simulink model "Quadrotor"  (R2022b)
settings: Solver=FixedStepAuto  StartTime=0.0  StopTime=1000  FixedStep=0.0005  RelTol=1e-3
model workspace (MAT data in the model file):
  b = 0.000142
  g = 9.8
  m = 1
undefined symbols (not defined in the file): Pitch, Roll, X, Y, Yaw, Z
libraries: simulink x12, slpidlib x9, sharedtransform x1, uavutilslib x1, aerolibanim x1
(part 2 of 3)

== system Quadrotor/Attitude Loop(PD)/P&R ==
  Pitch_d : Inport
  Roll_d : Inport  Port=2
  Pitch : Inport  Port=3
  Roll : Inport  Port=4
  PID Controller P : slpidlib/PID Controller  Controller=PD  Form=Parallel  TimeDomain=Continuous-time  UseExternalTs=off  SampleTime=-1  IntegratorMethod=Forward Euler  FilterMethod=Forward Euler  ControllerParametersSource=internal  P=0.002  I=1.51679966097293e-05  UseKiTs=off  D=0.004  N=3.58143563707461  UseFilter=on  TunerSelectOption=Transfer Function Based (PID Tuner App)  InitialConditionSource=internal  InitialConditionForIntegrator=0  InitialConditionForFilter=0  DifferentiatorICPrevScaledInput=0  ExternalReset=none  TrackingMode=off  Kt=1  LimitOutput=off  SatLimitsSource=internal  UpperSaturationLimit=inf  LowerSaturationLimit=-inf  LinearizeAsGain=on  AntiWindupMode=none  Kb=1  LimitIntegrator=off  UpperIntegratorSaturationLimit=inf  LowerIntegratorSaturationLimit=-inf  POutMin=[]  POutMax=[]  IOutMin=[]  IOutMax=[]  DOutMin=[]  DOutMax=[]  NOutMin=[]  NOutMax=[]  SumOutMin=[]  SumOutMax=[]  SaturationOutMin=[]  SaturationOutMax=[]  PParamMin=[]  PParamMax=[]  IParamMin=[]  IParamMax=[]  DParamMin=[]  DParamMax=[]  NParamMin=[]  NParamMax=[]  KbParamMin=[]  KbParamMax=[]  KtParamMin=[]  KtParamMax=[]  KbOutMin=[]  KbOutMax=[]  KtOutMin=[]  KtOutMax=[]  IntegratorOutMin=[]  IntegratorOutMax=[]  FilterOutMin=[]  FilterOutMax=[]  SumI1OutMin=[]  SumI1OutMax=[]  SumI2OutMin=[]  SumI2OutMax=[]  SumI3OutMin=[]  SumI3OutMax=[]  SumI4OutMin=[]  SumI4OutMax=[]  SumDOutMin=[]  SumDOutMax=[]  DifferentiatorOutMin=[]  DifferentiatorOutMax=[]  FilterDiffOutCoefMin=[]  FilterDiffOutCoefMax=[]  ReciprocalOutMin=[]  ReciprocalOutMax=[]  SumDenOutMin=[]  SumDenOutMax=[]  SumNumOutMin=[]  SumNumOutMax=[]  DivideOutMin=[]  DivideOutMax=[]  UdiffTsProdOutMin=[]  UdiffTsProdOutMax=[]  NTsProdOutMin=[]  NTsProdOutMax=[]  UintegralTsProdOutMin=[]  UintegralTsProdOutMax=[]  UngainTsProdOutMin=[]  UngainTsProdOutMax=[]  ClampingZeroOutDataTypeStr=Inherit: Inherit via back propagation  ClampingZeroOutMin=[]  ClampingZeroOutMax=[]  FilterDenConstantOutDataTypeStr=Inherit: Inherit via back propagation  FilterDenConstantOutMin=[]  FilterDenConstantOutMax=[]  PCopyOutDataTypeStr=Inherit: Inherit via back propagation  PCopyOutMin=[]  PCopyOutMax=[]  NCopyOutDataTypeStr=Inherit: Inherit via back propagation  NCopyOutMin=[]  NCopyOutMax=[]  IntegratorContinuousStateAttributes=''  IntegratorStateMustResolveToSignalObject=off  IntegratorRTWStateStorageClass=Auto  FilterContinuousStateAttributes=''  FilterStateMustResolveToSignalObject=off  FilterRTWStateStorageClass=Auto  ParallelPVariant=InternalParameters  IdealPVariant=Disabled  IVariant=Disabled  DVariant=InternalParameters  IntegratorVariant=Disabled  SatVariant=Disabled  AWVariant=Disabled  PCopyVariant=Disabled  TRVariant=Disabled  FdbkBlocksVariant=Forward  IdealPFdbkVariant=Disabled  SatFdbkVariant=Disabled  DerivativeFilterVariant=ContFilter  NVariant=InternalParameters  NCopyVariant=Disabled  FilterICVariant=InternalICsFilter  IntegratorICVariant=Disabled  ExternalResetVariant=Disabled  TRSumVariant=Passthrough  SumFdbkVariant=Disabled  SumVariant=Sum_PD  TsampFilterVariant=InternalTs  TsampNgainVariant=Passthrough  TsampIntegralVariant=Disabled_SignalSpec  ExternalSaturationOutDataTypeStr=Inherit: Same as second input
  PID Controller R : slpidlib/PID Controller  Controller=PD  Form=Parallel  TimeDomain=Continuous-time  UseExternalTs=off  SampleTime=-1  IntegratorMethod=Forward Euler  FilterMethod=Forward Euler  ControllerParametersSource=internal  P=0.000517944009365722  I=2.09015293720685e-05  UseKiTs=off  D=0.0031516571893313  N=4.69883432592557  UseFilter=on  TunerSelectOption=Transfer Function Based (PID Tuner App)  InitialConditionSource=internal  InitialConditionForIntegrator=0  InitialConditionForFilter=0  DifferentiatorICPrevScaledInput=0  ExternalReset=none  TrackingMode=off  Kt=1  LimitOutput=off  SatLimitsSource=internal  UpperSaturationLimit=inf  LowerSaturationLimit=-inf  LinearizeAsGain=on  AntiWindupMode=none  Kb=1  LimitIntegrator=off  UpperIntegratorSaturationLimit=inf  LowerIntegratorSaturationLimit=-inf  POutMin=[]  POutMax=[]  IOutMin=[]  IOutMax=[]  DOutMin=[]  DOutMax=[]  NOutMin=[]  NOutMax=[]  SumOutMin=[]  SumOutMax=[]  SaturationOutMin=[]  SaturationOutMax=[]  PParamMin=[]  PParamMax=[]  IParamMin=[]  IParamMax=[]  DParamMin=[]  DParamMax=[]  NParamMin=[]  NParamMax=[]  KbParamMin=[]  KbParamMax=[]  KtParamMin=[]  KtParamMax=[]  KbOutMin=[]  KbOutMax=[]  KtOutMin=[]  KtOutMax=[]  IntegratorOutMin=[]  IntegratorOutMax=[]  FilterOutMin=[]  FilterOutMax=[]  SumI1OutMin=[]  SumI1OutMax=[]  SumI2OutMin=[]  SumI2OutMax=[]  SumI3OutMin=[]  SumI3OutMax=[]  SumI4OutMin=[]  SumI4OutMax=[]  SumDOutMin=[]  SumDOutMax=[]  DifferentiatorOutMin=[]  DifferentiatorOutMax=[]  FilterDiffOutCoefMin=[]  FilterDiffOutCoefMax=[]  ReciprocalOutMin=[]  ReciprocalOutMax=[]  SumDenOutMin=[]  SumDenOutMax=[]  SumNumOutMin=[]  SumNumOutMax=[]  DivideOutMin=[]  DivideOutMax=[]  UdiffTsProdOutMin=[]  UdiffTsProdOutMax=[]  NTsProdOutMin=[]  NTsProdOutMax=[]  UintegralTsProdOutMin=[]  UintegralTsProdOutMax=[]  UngainTsProdOutMin=[]  UngainTsProdOutMax=[]  ClampingZeroOutDataTypeStr=Inherit: Inherit via back propagation  ClampingZeroOutMin=[]  ClampingZeroOutMax=[]  FilterDenConstantOutDataTypeStr=Inherit: Inherit via back propagation  FilterDenConstantOutMin=[]  FilterDenConstantOutMax=[]  PCopyOutDataTypeStr=Inherit: Inherit via back propagation  PCopyOutMin=[]  PCopyOutMax=[]  NCopyOutDataTypeStr=Inherit: Inherit via back propagation  NCopyOutMin=[]  NCopyOutMax=[]  IntegratorContinuousStateAttributes=''  IntegratorStateMustResolveToSignalObject=off  IntegratorRTWStateStorageClass=Auto  FilterContinuousStateAttributes=''  FilterStateMustResolveToSignalObject=off  FilterRTWStateStorageClass=Auto  ParallelPVariant=InternalParameters  IdealPVariant=Disabled  IVariant=Disabled  DVariant=InternalParameters  IntegratorVariant=Disabled  SatVariant=Disabled  AWVariant=Disabled  PCopyVariant=Disabled  TRVariant=Disabled  FdbkBlocksVariant=Forward  IdealPFdbkVariant=Disabled  SatFdbkVariant=Disabled  DerivativeFilterVariant=ContFilter  NVariant=InternalParameters  NCopyVariant=Disabled  FilterICVariant=InternalICsFilter  IntegratorICVariant=Disabled  ExternalResetVariant=Disabled  TRSumVariant=Passthrough  SumFdbkVariant=Disabled  SumVariant=Sum_PD  TsampFilterVariant=InternalTs  TsampNgainVariant=Passthrough  TsampIntegralVariant=Disabled_SignalSpec  ExternalSaturationOutDataTypeStr=Inherit: Same as second input
  Sum5 : Sum  Inputs=|+-
  Sum6 : Sum  Inputs=|+-
  U3 : Outport
  U2 : Outport  Port=2
  wires:
  PID Controller P/1 -> U3/1
  Pitch/1 -> Sum5/2
  Sum6/1 -> PID Controller R/1
  Sum5/1 -> PID Controller P/1
  Roll/1 -> Sum6/2
  PID Controller R/1 -> U2/1
  Pitch_d/1 -> Sum5/1
  Roll_d/1 -> Sum6/1

== system Quadrotor/Attitude Loop(PD)/yaw ==
  Yaw_d : Inport
  Yaw : Inport  Port=2
  PID Controller Y : slpidlib/PID Controller  Controller=PD  Form=Parallel  TimeDomain=Continuous-time  UseExternalTs=off  SampleTime=-1  IntegratorMethod=Forward Euler  FilterMethod=Forward Euler  ControllerParametersSource=internal  P=0.00070917828540938  I=0  UseKiTs=off  D=0.00337767414842328  N=2.26407668868773  UseFilter=on  TunerSelectOption=Transfer Function Based (PID Tuner App)  InitialConditionSource=internal  InitialConditionForIntegrator=0  InitialConditionForFilter=0  DifferentiatorICPrevScaledInput=0  ExternalReset=none  TrackingMode=off  Kt=1  LimitOutput=off  SatLimitsSource=internal  UpperSaturationLimit=inf  LowerSaturationLimit=-inf  LinearizeAsGain=on  AntiWindupMode=none  Kb=1  LimitIntegrator=off  UpperIntegratorSaturationLimit=inf  LowerIntegratorSaturationLimit=-inf  POutMin=[]  POutMax=[]  IOutMin=[]  IOutMax=[]  DOutMin=[]  DOutMax=[]  NOutMin=[]  NOutMax=[]  SumOutMin=[]  SumOutMax=[]  SaturationOutMin=[]  SaturationOutMax=[]  PParamMin=[]  PParamMax=[]  IParamMin=[]  IParamMax=[]  DParamMin=[]  DParamMax=[]  NParamMin=[]  NParamMax=[]  KbParamMin=[]  KbParamMax=[]  KtParamMin=[]  KtParamMax=[]  KbOutMin=[]  KbOutMax=[]  KtOutMin=[]  KtOutMax=[]  IntegratorOutMin=[]  IntegratorOutMax=[]  FilterOutMin=[]  FilterOutMax=[]  SumI1OutMin=[]  SumI1OutMax=[]  SumI2OutMin=[]  SumI2OutMax=[]  SumI3OutMin=[]  SumI3OutMax=[]  SumI4OutMin=[]  SumI4OutMax=[]  SumDOutMin=[]  SumDOutMax=[]  DifferentiatorOutMin=[]  DifferentiatorOutMax=[]  FilterDiffOutCoefMin=[]  FilterDiffOutCoefMax=[]  ReciprocalOutMin=[]  ReciprocalOutMax=[]  SumDenOutMin=[]  SumDenOutMax=[]  SumNumOutMin=[]  SumNumOutMax=[]  DivideOutMin=[]  DivideOutMax=[]  UdiffTsProdOutMin=[]  UdiffTsProdOutMax=[]  NTsProdOutMin=[]  NTsProdOutMax=[]  UintegralTsProdOutMin=[]  UintegralTsProdOutMax=[]  UngainTsProdOutMin=[]  UngainTsProdOutMax=[]  ClampingZeroOutDataTypeStr=Inherit: Inherit via back propagation  ClampingZeroOutMin=[]  ClampingZeroOutMax=[]  FilterDenConstantOutDataTypeStr=Inherit: Inherit via back propagation  FilterDenConstantOutMin=[]  FilterDenConstantOutMax=[]  PCopyOutDataTypeStr=Inherit: Inherit via back propagation  PCopyOutMin=[]  PCopyOutMax=[]  NCopyOutDataTypeStr=Inherit: Inherit via back propagation  NCopyOutMin=[]  NCopyOutMax=[]  IntegratorContinuousStateAttributes=''  IntegratorStateMustResolveToSignalObject=off  IntegratorRTWStateStorageClass=Auto  FilterContinuousStateAttributes=''  FilterStateMustResolveToSignalObject=off  FilterRTWStateStorageClass=Auto  ParallelPVariant=InternalParameters  IdealPVariant=Disabled  IVariant=Disabled  DVariant=InternalParameters  IntegratorVariant=Disabled  SatVariant=Disabled  AWVariant=Disabled  PCopyVariant=Disabled  TRVariant=Disabled  FdbkBlocksVariant=Forward  IdealPFdbkVariant=Disabled  SatFdbkVariant=Disabled  DerivativeFilterVariant=ContFilter  NVariant=InternalParameters  NCopyVariant=Disabled  FilterICVariant=InternalICsFilter  IntegratorICVariant=Disabled  ExternalResetVariant=Disabled  TRSumVariant=Passthrough  SumFdbkVariant=Disabled  SumVariant=Sum_PD  TsampFilterVariant=InternalTs  TsampNgainVariant=Passthrough  TsampIntegralVariant=Disabled_SignalSpec  ExternalSaturationOutDataTypeStr=Inherit: Same as second input
  Sum2 : Sum  Inputs=|+-
  U4 : Outport
  wires:
  Yaw/1 -> Sum2/2
  Sum2/1 -> PID Controller Y/1
  Yaw_d/1 -> Sum2/1
  PID Controller Y/1 -> U4/1

== system Quadrotor/Demand_LADRC/generate ==
  butterfly : Subsystem
  circle 500 : Subsystem
  ramp 30 : Subsystem
  screw 600 : Subsystem
  steady1 : Subsystem
  up 30 : Subsystem
  up : Outport
  ramp : Outport  Port=2
  circle : Outport  Port=3
  screw : Outport  Port=4
  butterfiy : Outport  Port=5
  steady : Outport  Port=6
  wires:
  screw 600/1(Out1) -> screw/1
  butterfly/1(Out1) -> butterfiy/1
  circle 500/1(Out1) -> circle/1
  ramp 30/1(Out1) -> ramp/1
  up 30/1(Out1) -> up/1
  steady1/1(Out1) -> steady/1

== system Quadrotor/Demand_LADRC/out ==
  In1 : Inport
  Bus Selector : BusSelector  OutputSignals=signal1,signal2,signal3,signal4
  To Workspace : ToWorkspace  VariableName=demand1  SampleTime=-1
  X_d : Outport
  Y_d : Outport  Port=2
  Z_d : Outport  Port=3
  Yaw_d : Outport  Port=4
  wires:
  Bus Selector/3 -> Z_d/1  "<signal3>"
  Bus Selector/2 -> Y_d/1  "<signal2>"
  Bus Selector/1 -> X_d/1  "<signal1>"
  Bus Selector/4 -> Yaw_d/1  "<signal4>"
  In1/1 -> To Workspace/1, Bus Selector/1

== system Quadrotor/Demand_PID/generate ==
  butterfly : Subsystem
  circle 500 : Subsystem
  ramp 30 : Subsystem
  screw 600 : Subsystem
  steady1 : Subsystem
  up 30 : Subsystem
  up : Outport
  ramp : Outport  Port=2
  circle : Outport  Port=3
  screw : Outport  Port=4
  butterfiy : Outport  Port=5
  steady : Outport  Port=6
  wires:
  screw 600/1(Out1) -> screw/1
  butterfly/1(Out1) -> butterfiy/1
  circle 500/1(Out1) -> circle/1
  ramp 30/1(Out1) -> ramp/1
  up 30/1(Out1) -> up/1
  steady1/1(Out1) -> steady/1

== system Quadrotor/Demand_PID/out ==
  In1 : Inport
  Bus Selector : BusSelector  OutputSignals=signal1,signal2,signal3,signal4
  To Workspace : ToWorkspace  VariableName=demand  SampleTime=-1
  X_d : Outport
  Y_d : Outport  Port=2
  Z_d : Outport  Port=3
  Yaw_d : Outport  Port=4
  wires:
  Bus Selector/3 -> Z_d/1  "<signal3>"
  Bus Selector/2 -> Y_d/1  "<signal2>"
  Bus Selector/1 -> X_d/1  "<signal1>"
  Bus Selector/4 -> Yaw_d/1  "<signal4>"
  In1/1 -> To Workspace/1, Bus Selector/1

== system Quadrotor/Formation Control/height ==
  Z_d : Inport
  Z : Inport  Port=2
  Constant : Constant  Value=g
  PID Controller Z : slpidlib/PID Controller  Controller=PID  Form=Parallel  TimeDomain=Discrete-time  UseExternalTs=off  SampleTime=-1  IntegratorMethod=Forward Euler  FilterMethod=Forward Euler  ControllerParametersSource=internal  P=3.53804542303513  I=0.723013447865675  UseKiTs=off  D=4.25131927818495  N=23.8074436453229  UseFilter=on  TunerSelectOption=Transfer Function Based (PID Tuner App)  InitialConditionSource=internal  InitialConditionForIntegrator=0  InitialConditionForFilter=0  DifferentiatorICPrevScaledInput=0  ExternalReset=none  TrackingMode=off  Kt=1  LimitOutput=off  SatLimitsSource=internal  UpperSaturationLimit=inf  LowerSaturationLimit=-inf  LinearizeAsGain=on  AntiWindupMode=none  Kb=1  LimitIntegrator=off  UpperIntegratorSaturationLimit=inf  LowerIntegratorSaturationLimit=-inf  POutMin=[]  POutMax=[]  IOutMin=[]  IOutMax=[]  DOutMin=[]  DOutMax=[]  NOutMin=[]  NOutMax=[]  SumOutMin=[]  SumOutMax=[]  SaturationOutMin=[]  SaturationOutMax=[]  PParamMin=[]  PParamMax=[]  IParamMin=[]  IParamMax=[]  DParamMin=[]  DParamMax=[]  NParamMin=[]  NParamMax=[]  KbParamMin=[]  KbParamMax=[]  KtParamMin=[]  KtParamMax=[]  KbOutMin=[]  KbOutMax=[]  KtOutMin=[]  KtOutMax=[]  IntegratorOutMin=[]  IntegratorOutMax=[]  FilterOutMin=[]  FilterOutMax=[]  SumI1OutMin=[]  SumI1OutMax=[]  SumI2OutMin=[]  SumI2OutMax=[]  SumI3OutMin=[]  SumI3OutMax=[]  SumI4OutMin=[]  SumI4OutMax=[]  SumDOutMin=[]  SumDOutMax=[]  DifferentiatorOutMin=[]  DifferentiatorOutMax=[]  FilterDiffOutCoefMin=[]  FilterDiffOutCoefMax=[]  ReciprocalOutMin=[]  ReciprocalOutMax=[]  SumDenOutMin=[]  SumDenOutMax=[]  SumNumOutMin=[]  SumNumOutMax=[]  DivideOutMin=[]  DivideOutMax=[]  UdiffTsProdOutMin=[]  UdiffTsProdOutMax=[]  NTsProdOutMin=[]  NTsProdOutMax=[]  UintegralTsProdOutMin=[]  UintegralTsProdOutMax=[]  UngainTsProdOutMin=[]  UngainTsProdOutMax=[]  ClampingZeroOutDataTypeStr=Inherit: Inherit via back propagation  ClampingZeroOutMin=[]  ClampingZeroOutMax=[]  FilterDenConstantOutDataTypeStr=Inherit: Inherit via back propagation  FilterDenConstantOutMin=[]  FilterDenConstantOutMax=[]  PCopyOutDataTypeStr=Inherit: Inherit via back propagation  PCopyOutMin=[]  PCopyOutMax=[]  NCopyOutDataTypeStr=Inherit: Inherit via back propagation  NCopyOutMin=[]  NCopyOutMax=[]  IntegratorContinuousStateAttributes=''  IntegratorStateMustResolveToSignalObject=off  IntegratorRTWStateStorageClass=Auto  FilterContinuousStateAttributes=''  FilterStateMustResolveToSignalObject=off  FilterRTWStateStorageClass=Auto  ParallelPVariant=InternalParameters  IdealPVariant=Disabled  IVariant=InternalParameters  DVariant=InternalParameters  IntegratorVariant=Discrete  SatVariant=Disabled  AWVariant=Passthrough  PCopyVariant=Disabled  TRVariant=Disabled  FdbkBlocksVariant=Forward  IdealPFdbkVariant=Disabled  SatFdbkVariant=Disabled  DerivativeFilterVariant=ForwardEulerFilter  NVariant=InternalParameters  NCopyVariant=Disabled  FilterICVariant=InternalICsFilter  IntegratorICVariant=InternalICs  ExternalResetVariant=Disabled  TRSumVariant=Passthrough  SumFdbkVariant=Disabled  SumVariant=Sum_PID  TsampFilterVariant=InternalTs  TsampNgainVariant=Passthrough  TsampIntegralVariant=Passthrough  ExternalSaturationOutDataTypeStr=Inherit: Same as second input
  Sum : Sum  Inputs=-+|
  Sum1 : Sum  Inputs=++|
  Uz+g : Outport
  wires:
  Z/1 -> Sum/1
  Z_d/1 -> Sum/2
  Constant/1 -> Sum1/1
  Sum/1 -> PID Controller Z/1
  PID Controller Z/1 -> Sum1/2
  Sum1/1 -> Uz+g/1

== system Quadrotor/Formation Control/location  ==
  X_d : Inport
  Y_d : Inport  Port=2
  X : Inport  Port=3
  Y : Inport  Port=4
  Derivative{,1..3} (4 alike) : Derivative
  PID Controller X : slpidlib/PID Controller  Controller=PD  Form=Parallel  TimeDomain=Discrete-time  UseExternalTs=off  SampleTime=-1  IntegratorMethod=Forward Euler  FilterMethod=Forward Euler  ControllerParametersSource=internal  P=0.01  I=1.32852953365654e-05  UseKiTs=off  D=0.16  N=9.20175473255031  UseFilter=on  TunerSelectOption=Transfer Function Based (PID Tuner App)  InitialConditionSource=internal  InitialConditionForIntegrator=0  InitialConditionForFilter=0  DifferentiatorICPrevScaledInput=0  ExternalReset=none  TrackingMode=off  Kt=1  LimitOutput=off  SatLimitsSource=internal  UpperSaturationLimit=inf  LowerSaturationLimit=-inf  LinearizeAsGain=on  AntiWindupMode=none  Kb=1  LimitIntegrator=off  UpperIntegratorSaturationLimit=inf  LowerIntegratorSaturationLimit=-inf  POutMin=[]  POutMax=[]  IOutMin=[]  IOutMax=[]  DOutMin=[]  DOutMax=[]  NOutMin=[]  NOutMax=[]  SumOutMin=[]  SumOutMax=[]  SaturationOutMin=[]  SaturationOutMax=[]  PParamMin=[]  PParamMax=[]  IParamMin=[]  IParamMax=[]  DParamMin=[]  DParamMax=[]  NParamMin=[]  NParamMax=[]  KbParamMin=[]  KbParamMax=[]  KtParamMin=[]  KtParamMax=[]  KbOutMin=[]  KbOutMax=[]  KtOutMin=[]  KtOutMax=[]  IntegratorOutMin=[]  IntegratorOutMax=[]  FilterOutMin=[]  FilterOutMax=[]  SumI1OutMin=[]  SumI1OutMax=[]  SumI2OutMin=[]  SumI2OutMax=[]  SumI3OutMin=[]  SumI3OutMax=[]  SumI4OutMin=[]  SumI4OutMax=[]  SumDOutMin=[]  SumDOutMax=[]  DifferentiatorOutMin=[]  DifferentiatorOutMax=[]  FilterDiffOutCoefMin=[]  FilterDiffOutCoefMax=[]  ReciprocalOutMin=[]  ReciprocalOutMax=[]  SumDenOutMin=[]  SumDenOutMax=[]  SumNumOutMin=[]  SumNumOutMax=[]  DivideOutMin=[]  DivideOutMax=[]  UdiffTsProdOutMin=[]  UdiffTsProdOutMax=[]  NTsProdOutMin=[]  NTsProdOutMax=[]  UintegralTsProdOutMin=[]  UintegralTsProdOutMax=[]  UngainTsProdOutMin=[]  UngainTsProdOutMax=[]  ClampingZeroOutDataTypeStr=Inherit: Inherit via back propagation  ClampingZeroOutMin=[]  ClampingZeroOutMax=[]  FilterDenConstantOutDataTypeStr=Inherit: Inherit via back propagation  FilterDenConstantOutMin=[]  FilterDenConstantOutMax=[]  PCopyOutDataTypeStr=Inherit: Inherit via back propagation  PCopyOutMin=[]  PCopyOutMax=[]  NCopyOutDataTypeStr=Inherit: Inherit via back propagation  NCopyOutMin=[]  NCopyOutMax=[]  IntegratorContinuousStateAttributes=''  IntegratorStateMustResolveToSignalObject=off  IntegratorRTWStateStorageClass=Auto  FilterContinuousStateAttributes=''  FilterStateMustResolveToSignalObject=off  FilterRTWStateStorageClass=Auto  ParallelPVariant=InternalParameters  IdealPVariant=Disabled  IVariant=Disabled  DVariant=InternalParameters  IntegratorVariant=Disabled  SatVariant=Disabled  AWVariant=Disabled  PCopyVariant=Disabled  TRVariant=Disabled  FdbkBlocksVariant=Forward  IdealPFdbkVariant=Disabled  SatFdbkVariant=Disabled  DerivativeFilterVariant=ForwardEulerFilter  NVariant=InternalParameters  NCopyVariant=Disabled  FilterICVariant=InternalICsFilter  IntegratorICVariant=Disabled  ExternalResetVariant=Disabled  TRSumVariant=Passthrough  SumFdbkVariant=Disabled  SumVariant=Sum_PD  TsampFilterVariant=InternalTs  TsampNgainVariant=Passthrough  TsampIntegralVariant=Disabled_SignalSpec  ExternalSaturationOutDataTypeStr=Inherit: Same as second input
  PID Controller Y : slpidlib/PID Controller  Controller=PD  Form=Parallel  TimeDomain=Discrete-time  UseExternalTs=off  SampleTime=-1  IntegratorMethod=Forward Euler  FilterMethod=Forward Euler  ControllerParametersSource=internal  P=0.01  I=2.10922571180575e-05  UseKiTs=off  D=0.16  N=9.20175473255031  UseFilter=on  TunerSelectOption=Transfer Function Based (PID Tuner App)  InitialConditionSource=internal  InitialConditionForIntegrator=0  InitialConditionForFilter=0  DifferentiatorICPrevScaledInput=0  ExternalReset=none  TrackingMode=off  Kt=1  LimitOutput=off  SatLimitsSource=internal  UpperSaturationLimit=inf  LowerSaturationLimit=-inf  LinearizeAsGain=on  AntiWindupMode=none  Kb=1  LimitIntegrator=off  UpperIntegratorSaturationLimit=inf  LowerIntegratorSaturationLimit=-inf  POutMin=[]  POutMax=[]  IOutMin=[]  IOutMax=[]  DOutMin=[]  DOutMax=[]  NOutMin=[]  NOutMax=[]  SumOutMin=[]  SumOutMax=[]  SaturationOutMin=[]  SaturationOutMax=[]  PParamMin=[]  PParamMax=[]  IParamMin=[]  IParamMax=[]  DParamMin=[]  DParamMax=[]  NParamMin=[]  NParamMax=[]  KbParamMin=[]  KbParamMax=[]  KtParamMin=[]  KtParamMax=[]  KbOutMin=[]  KbOutMax=[]  KtOutMin=[]  KtOutMax=[]  IntegratorOutMin=[]  IntegratorOutMax=[]  FilterOutMin=[]  FilterOutMax=[]  SumI1OutMin=[]  SumI1OutMax=[]  SumI2OutMin=[]  SumI2OutMax=[]  SumI3OutMin=[]  SumI3OutMax=[]  SumI4OutMin=[]  SumI4OutMax=[]  SumDOutMin=[]  SumDOutMax=[]  DifferentiatorOutMin=[]  DifferentiatorOutMax=[]  FilterDiffOutCoefMin=[]  FilterDiffOutCoefMax=[]  ReciprocalOutMin=[]  ReciprocalOutMax=[]  SumDenOutMin=[]  SumDenOutMax=[]  SumNumOutMin=[]  SumNumOutMax=[]  DivideOutMin=[]  DivideOutMax=[]  UdiffTsProdOutMin=[]  UdiffTsProdOutMax=[]  NTsProdOutMin=[]  NTsProdOutMax=[]  UintegralTsProdOutMin=[]  UintegralTsProdOutMax=[]  UngainTsProdOutMin=[]  UngainTsProdOutMax=[]  ClampingZeroOutDataTypeStr=Inherit: Inherit via back propagation  ClampingZeroOutMin=[]  ClampingZeroOutMax=[]  FilterDenConstantOutDataTypeStr=Inherit: Inherit via back propagation  FilterDenConstantOutMin=[]  FilterDenConstantOutMax=[]  PCopyOutDataTypeStr=Inherit: Inherit via back propagation  PCopyOutMin=[]  PCopyOutMax=[]  NCopyOutDataTypeStr=Inherit: Inherit via back propagation  NCopyOutMin=[]  NCopyOutMax=[]  IntegratorContinuousStateAttributes=''  IntegratorStateMustResolveToSignalObject=off  IntegratorRTWStateStorageClass=Auto  FilterContinuousStateAttributes=''  FilterStateMustResolveToSignalObject=off  FilterRTWStateStorageClass=Auto  ParallelPVariant=InternalParameters  IdealPVariant=Disabled  IVariant=Disabled  DVariant=InternalParameters  IntegratorVariant=Disabled  SatVariant=Disabled  AWVariant=Disabled  PCopyVariant=Disabled  TRVariant=Disabled  FdbkBlocksVariant=Forward  IdealPFdbkVariant=Disabled  SatFdbkVariant=Disabled  DerivativeFilterVariant=ForwardEulerFilter  NVariant=InternalParameters  NCopyVariant=Disabled  FilterICVariant=InternalICsFilter  IntegratorICVariant=Disabled  ExternalResetVariant=Disabled  TRSumVariant=Passthrough  SumFdbkVariant=Disabled  SumVariant=Sum_PD  TsampFilterVariant=InternalTs  TsampNgainVariant=Passthrough  TsampIntegralVariant=Disabled_SignalSpec  ExternalSaturationOutDataTypeStr=Inherit: Same as second input
  Sum1 : Sum  Inputs=|++
  Sum2 : Sum  Inputs=|++
  Sum3 : Sum  Inputs=-+|
  Sum4 : Sum  Inputs=-+|
  X' : Outport
  Y' : Outport  Port=2
  wires:
  X_d/1 -> Derivative/1, Sum4/2
  Y_d/1 -> Derivative3/1, Sum3/2
  X/1 -> Sum4/1
  Y/1 -> Sum3/1
  Sum4/1 -> PID Controller X/1
  Sum3/1 -> PID Controller Y/1
  Derivative/1 -> Derivative1/1
  PID Controller X/1 -> Sum1/1
  Sum1/1 -> X'/1
  Derivative1/1 -> Sum1/2
  Derivative3/1 -> Derivative2/1
  Derivative2/1 -> Sum2/2
  PID Controller Y/1 -> Sum2/1
  Sum2/1 -> Y'/1

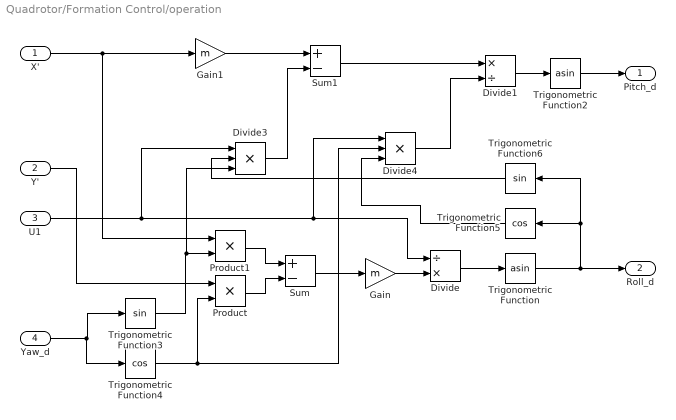
== system Quadrotor/Formation Control/operation ==
  X' : Inport
  Y' : Inport  Port=2
  U1 : Inport  Port=3
  Yaw_d : Inport  Port=4
  Divide : Product  Inputs=/*
  Divide1 : Product  Inputs=*/
  Divide3 : Product  Inputs=***
  Divide4 : Product  Inputs=***
  Gain : Gain  Gain=m
  Gain1 : Gain  Gain=m
  Product : Product
  Product1 : Product
  Sum : Sum  Inputs=+-
  Sum1 : Sum  Inputs=+-
  Trigonometric Function : Trigonometry  Operator=asin
  Trigonometric Function2 : Trigonometry  Operator=asin
  Trigonometric Function3 : Trigonometry
  Trigonometric Function4 : Trigonometry  Operator=cos
  Trigonometric Function5 : Trigonometry  Operator=cos
  Trigonometric Function6 : Trigonometry
  Pitch_d : Outport
  Roll_d : Outport  Port=2
  wires:
  Yaw_d/1 -> Trigonometric Function4/1, Trigonometric Function3/1
  X'/1 -> Gain1/1, Product1/1
  Trigonometric Function3/1 -> Divide3/3, Product1/2
  Y'/1 -> Product/1
  Trigonometric Function4/1 -> Product/2, Divide4/2
  Product1/1 -> Sum/1
  Product/1 -> Sum/2
  Sum/1 -> Gain/1
  Divide/1 -> Trigonometric Function/1
  Trigonometric Function/1 -> Trigonometric Function5/1, Trigonometric Function6/1, Roll_d/1
  Gain1/1 -> Sum1/1
  Gain/1 -> Divide/2
  U1/1 -> Divide3/1, Divide4/1, Divide/1
  Trigonometric Function6/1 -> Divide3/2
  Divide3/1 -> Sum1/2
  Sum1/1 -> Divide1/1
  Trigonometric Function5/1 -> Divide4/3
  Divide4/1 -> Divide1/2
  Divide1/1 -> Trigonometric Function2/1
  Trigonometric Function2/1 -> Pitch_d/1

== system Quadrotor/Formation Control/sum ==
  Uz+g : Inport
  Ux : Inport  Port=2
  Uy : Inport  Port=3
  Gain : Gain  Gain=m
  Square : Math  Operator=square
  Square Root : Sqrt
  Square1 : Math  Operator=square
  Square2 : Math  Operator=square
  Sum : Sum  Inputs=+++
  U1 : Outport
  wires:
  Ux/1 -> Square/1
  Uz+g/1 -> Square2/1
  Uy/1 -> Square1/1
  Square/1 -> Sum/1
  Square1/1 -> Sum/2
  Square2/1 -> Sum/3
  Sum/1 -> Square Root/1
  Gain/1 -> U1/1
  Square Root/1 -> Gain/1

== system Quadrotor/Formation Control(PID)/height ==
  Z_d : Inport
  Z : Inport  Port=2
  Constant : Constant  Value=g
  PID Controller Z : slpidlib/PID Controller  Controller=PID  Form=Parallel  TimeDomain=Continuous-time  UseExternalTs=off  SampleTime=-1  IntegratorMethod=Forward Euler  FilterMethod=Forward Euler  ControllerParametersSource=internal  P=3.53804542303513  I=0.723013447865675  UseKiTs=off  D=4.25131927818495  N=23.8074436453229  UseFilter=on  TunerSelectOption=Transfer Function Based (PID Tuner App)  InitialConditionSource=internal  InitialConditionForIntegrator=0  InitialConditionForFilter=0  DifferentiatorICPrevScaledInput=0  ExternalReset=none  TrackingMode=off  Kt=1  LimitOutput=off  SatLimitsSource=internal  UpperSaturationLimit=inf  LowerSaturationLimit=-inf  LinearizeAsGain=on  AntiWindupMode=none  Kb=1  LimitIntegrator=off  UpperIntegratorSaturationLimit=inf  LowerIntegratorSaturationLimit=-inf  POutMin=[]  POutMax=[]  IOutMin=[]  IOutMax=[]  DOutMin=[]  DOutMax=[]  NOutMin=[]  NOutMax=[]  SumOutMin=[]  SumOutMax=[]  SaturationOutMin=[]  SaturationOutMax=[]  PParamMin=[]  PParamMax=[]  IParamMin=[]  IParamMax=[]  DParamMin=[]  DParamMax=[]  NParamMin=[]  NParamMax=[]  KbParamMin=[]  KbParamMax=[]  KtParamMin=[]  KtParamMax=[]  KbOutMin=[]  KbOutMax=[]  KtOutMin=[]  KtOutMax=[]  IntegratorOutMin=[]  IntegratorOutMax=[]  FilterOutMin=[]  FilterOutMax=[]  SumI1OutMin=[]  SumI1OutMax=[]  SumI2OutMin=[]  SumI2OutMax=[]  SumI3OutMin=[]  SumI3OutMax=[]  SumI4OutMin=[]  SumI4OutMax=[]  SumDOutMin=[]  SumDOutMax=[]  DifferentiatorOutMin=[]  DifferentiatorOutMax=[]  FilterDiffOutCoefMin=[]  FilterDiffOutCoefMax=[]  ReciprocalOutMin=[]  ReciprocalOutMax=[]  SumDenOutMin=[]  SumDenOutMax=[]  SumNumOutMin=[]  SumNumOutMax=[]  DivideOutMin=[]  DivideOutMax=[]  UdiffTsProdOutMin=[]  UdiffTsProdOutMax=[]  NTsProdOutMin=[]  NTsProdOutMax=[]  UintegralTsProdOutMin=[]  UintegralTsProdOutMax=[]  UngainTsProdOutMin=[]  UngainTsProdOutMax=[]  ClampingZeroOutDataTypeStr=Inherit: Inherit via back propagation  ClampingZeroOutMin=[]  ClampingZeroOutMax=[]  FilterDenConstantOutDataTypeStr=Inherit: Inherit via back propagation  FilterDenConstantOutMin=[]  FilterDenConstantOutMax=[]  PCopyOutDataTypeStr=Inherit: Inherit via back propagation  PCopyOutMin=[]  PCopyOutMax=[]  NCopyOutDataTypeStr=Inherit: Inherit via back propagation  NCopyOutMin=[]  NCopyOutMax=[]  IntegratorContinuousStateAttributes=''  IntegratorStateMustResolveToSignalObject=off  IntegratorRTWStateStorageClass=Auto  FilterContinuousStateAttributes=''  FilterStateMustResolveToSignalObject=off  FilterRTWStateStorageClass=Auto  ParallelPVariant=InternalParameters  IdealPVariant=Disabled  IVariant=InternalParameters  DVariant=InternalParameters  IntegratorVariant=Continuous  SatVariant=Disabled  AWVariant=Passthrough  PCopyVariant=Disabled  TRVariant=Disabled  FdbkBlocksVariant=Forward  IdealPFdbkVariant=Disabled  SatFdbkVariant=Disabled  DerivativeFilterVariant=ContFilter  NVariant=InternalParameters  NCopyVariant=Disabled  FilterICVariant=InternalICsFilter  IntegratorICVariant=InternalICs  ExternalResetVariant=Disabled  TRSumVariant=Passthrough  SumFdbkVariant=Disabled  SumVariant=Sum_PID  TsampFilterVariant=InternalTs  TsampNgainVariant=Passthrough  TsampIntegralVariant=Passthrough  ExternalSaturationOutDataTypeStr=Inherit: Same as second input
  Sum : Sum  Inputs=-+|
  Sum1 : Sum  Inputs=++|
  U1 : Outport
  wires:
  Z/1 -> Sum/1
  Z_d/1 -> Sum/2
  Constant/1 -> Sum1/1
  Sum/1 -> PID Controller Z/1
  PID Controller Z/1 -> Sum1/2
  Sum1/1 -> U1/1

== system Quadrotor/Formation Control(PID)/location  ==
  X_d : Inport
  Y_d : Inport  Port=2
  X : Inport  Port=3
  Y : Inport  Port=4
  Derivative{,1..3} (4 alike) : Derivative
  PID Controller X : slpidlib/PID Controller  Controller=PD  Form=Parallel  TimeDomain=Continuous-time  UseExternalTs=off  SampleTime=-1  IntegratorMethod=Forward Euler  FilterMethod=Forward Euler  ControllerParametersSource=internal  P=0.0025  I=1.32852953365654e-05  UseKiTs=off  D=0.13  N=0.173869187987419  UseFilter=on  TunerSelectOption=Transfer Function Based (PID Tuner App)  InitialConditionSource=internal  InitialConditionForIntegrator=0  InitialConditionForFilter=0  DifferentiatorICPrevScaledInput=0  ExternalReset=none  TrackingMode=off  Kt=1  LimitOutput=off  SatLimitsSource=internal  UpperSaturationLimit=inf  LowerSaturationLimit=-inf  LinearizeAsGain=on  AntiWindupMode=none  Kb=1  LimitIntegrator=off  UpperIntegratorSaturationLimit=inf  LowerIntegratorSaturationLimit=-inf  POutMin=[]  POutMax=[]  IOutMin=[]  IOutMax=[]  DOutMin=[]  DOutMax=[]  NOutMin=[]  NOutMax=[]  SumOutMin=[]  SumOutMax=[]  SaturationOutMin=[]  SaturationOutMax=[]  PParamMin=[]  PParamMax=[]  IParamMin=[]  IParamMax=[]  DParamMin=[]  DParamMax=[]  NParamMin=[]  NParamMax=[]  KbParamMin=[]  KbParamMax=[]  KtParamMin=[]  KtParamMax=[]  KbOutMin=[]  KbOutMax=[]  KtOutMin=[]  KtOutMax=[]  IntegratorOutMin=[]  IntegratorOutMax=[]  FilterOutMin=[]  FilterOutMax=[]  SumI1OutMin=[]  SumI1OutMax=[]  SumI2OutMin=[]  SumI2OutMax=[]  SumI3OutMin=[]  SumI3OutMax=[]  SumI4OutMin=[]  SumI4OutMax=[]  SumDOutMin=[]  SumDOutMax=[]  DifferentiatorOutMin=[]  DifferentiatorOutMax=[]  FilterDiffOutCoefMin=[]  FilterDiffOutCoefMax=[]  ReciprocalOutMin=[]  ReciprocalOutMax=[]  SumDenOutMin=[]  SumDenOutMax=[]  SumNumOutMin=[]  SumNumOutMax=[]  DivideOutMin=[]  DivideOutMax=[]  UdiffTsProdOutMin=[]  UdiffTsProdOutMax=[]  NTsProdOutMin=[]  NTsProdOutMax=[]  UintegralTsProdOutMin=[]  UintegralTsProdOutMax=[]  UngainTsProdOutMin=[]  UngainTsProdOutMax=[]  ClampingZeroOutDataTypeStr=Inherit: Inherit via back propagation  ClampingZeroOutMin=[]  ClampingZeroOutMax=[]  FilterDenConstantOutDataTypeStr=Inherit: Inherit via back propagation  FilterDenConstantOutMin=[]  FilterDenConstantOutMax=[]  PCopyOutDataTypeStr=Inherit: Inherit via back propagation  PCopyOutMin=[]  PCopyOutMax=[]  NCopyOutDataTypeStr=Inherit: Inherit via back propagation  NCopyOutMin=[]  NCopyOutMax=[]  IntegratorContinuousStateAttributes=''  IntegratorStateMustResolveToSignalObject=off  IntegratorRTWStateStorageClass=Auto  FilterContinuousStateAttributes=''  FilterStateMustResolveToSignalObject=off  FilterRTWStateStorageClass=Auto  ParallelPVariant=InternalParameters  IdealPVariant=Disabled  IVariant=Disabled  DVariant=InternalParameters  IntegratorVariant=Disabled  SatVariant=Disabled  AWVariant=Disabled  PCopyVariant=Disabled  TRVariant=Disabled  FdbkBlocksVariant=Forward  IdealPFdbkVariant=Disabled  SatFdbkVariant=Disabled  DerivativeFilterVariant=ContFilter  NVariant=InternalParameters  NCopyVariant=Disabled  FilterICVariant=InternalICsFilter  IntegratorICVariant=Disabled  ExternalResetVariant=Disabled  TRSumVariant=Passthrough  SumFdbkVariant=Disabled  SumVariant=Sum_PD  TsampFilterVariant=InternalTs  TsampNgainVariant=Passthrough  TsampIntegralVariant=Disabled_SignalSpec  ExternalSaturationOutDataTypeStr=Inherit: Same as second input
  PID Controller Y : slpidlib/PID Controller  Controller=PD  Form=Parallel  TimeDomain=Continuous-time  UseExternalTs=off  SampleTime=-1  IntegratorMethod=Forward Euler  FilterMethod=Forward Euler  ControllerParametersSource=internal  P=0.01  I=2.10922571180575e-05  UseKiTs=off  D=0.16  N=9.20175473255031  UseFilter=on  TunerSelectOption=Transfer Function Based (PID Tuner App)  InitialConditionSource=internal  InitialConditionForIntegrator=0  InitialConditionForFilter=0  DifferentiatorICPrevScaledInput=0  ExternalReset=none  TrackingMode=off  Kt=1  LimitOutput=off  SatLimitsSource=internal  UpperSaturationLimit=inf  LowerSaturationLimit=-inf  LinearizeAsGain=on  AntiWindupMode=none  Kb=1  LimitIntegrator=off  UpperIntegratorSaturationLimit=inf  LowerIntegratorSaturationLimit=-inf  POutMin=[]  POutMax=[]  IOutMin=[]  IOutMax=[]  DOutMin=[]  DOutMax=[]  NOutMin=[]  NOutMax=[]  SumOutMin=[]  SumOutMax=[]  SaturationOutMin=[]  SaturationOutMax=[]  PParamMin=[]  PParamMax=[]  IParamMin=[]  IParamMax=[]  DParamMin=[]  DParamMax=[]  NParamMin=[]  NParamMax=[]  KbParamMin=[]  KbParamMax=[]  KtParamMin=[]  KtParamMax=[]  KbOutMin=[]  KbOutMax=[]  KtOutMin=[]  KtOutMax=[]  IntegratorOutMin=[]  IntegratorOutMax=[]  FilterOutMin=[]  FilterOutMax=[]  SumI1OutMin=[]  SumI1OutMax=[]  SumI2OutMin=[]  SumI2OutMax=[]  SumI3OutMin=[]  SumI3OutMax=[]  SumI4OutMin=[]  SumI4OutMax=[]  SumDOutMin=[]  SumDOutMax=[]  DifferentiatorOutMin=[]  DifferentiatorOutMax=[]  FilterDiffOutCoefMin=[]  FilterDiffOutCoefMax=[]  ReciprocalOutMin=[]  ReciprocalOutMax=[]  SumDenOutMin=[]  SumDenOutMax=[]  SumNumOutMin=[]  SumNumOutMax=[]  DivideOutMin=[]  DivideOutMax=[]  UdiffTsProdOutMin=[]  UdiffTsProdOutMax=[]  NTsProdOutMin=[]  NTsProdOutMax=[]  UintegralTsProdOutMin=[]  UintegralTsProdOutMax=[]  UngainTsProdOutMin=[]  UngainTsProdOutMax=[]  ClampingZeroOutDataTypeStr=Inherit: Inherit via back propagation  ClampingZeroOutMin=[]  ClampingZeroOutMax=[]  FilterDenConstantOutDataTypeStr=Inherit: Inherit via back propagation  FilterDenConstantOutMin=[]  FilterDenConstantOutMax=[]  PCopyOutDataTypeStr=Inherit: Inherit via back propagation  PCopyOutMin=[]  PCopyOutMax=[]  NCopyOutDataTypeStr=Inherit: Inherit via back propagation  NCopyOutMin=[]  NCopyOutMax=[]  IntegratorContinuousStateAttributes=''  IntegratorStateMustResolveToSignalObject=off  IntegratorRTWStateStorageClass=Auto  FilterContinuousStateAttributes=''  FilterStateMustResolveToSignalObject=off  FilterRTWStateStorageClass=Auto  ParallelPVariant=InternalParameters  IdealPVariant=Disabled  IVariant=Disabled  DVariant=InternalParameters  IntegratorVariant=Disabled  SatVariant=Disabled  AWVariant=Disabled  PCopyVariant=Disabled  TRVariant=Disabled  FdbkBlocksVariant=Forward  IdealPFdbkVariant=Disabled  SatFdbkVariant=Disabled  DerivativeFilterVariant=ContFilter  NVariant=InternalParameters  NCopyVariant=Disabled  FilterICVariant=InternalICsFilter  IntegratorICVariant=Disabled  ExternalResetVariant=Disabled  TRSumVariant=Passthrough  SumFdbkVariant=Disabled  SumVariant=Sum_PD  TsampFilterVariant=InternalTs  TsampNgainVariant=Passthrough  TsampIntegralVariant=Disabled_SignalSpec  ExternalSaturationOutDataTypeStr=Inherit: Same as second input
  Sum3 : Sum  Inputs=-+|
  Sum4 : Sum  Inputs=-+|
  Sum7 : Sum  Inputs=|++
  Sum8 : Sum  Inputs=|++
  X' : Outport
  Y' : Outport  Port=2
  wires:
  Derivative2/1 -> Derivative3/1
  Sum8/1 -> Y'/1
  Derivative1/1 -> Sum7/2
  Derivative/1 -> Derivative1/1
  Derivative3/1 -> Sum8/2
  X_d/1 -> Sum4/2, Derivative/1
  Y_d/1 -> Sum3/2, Derivative2/1
  Sum4/1 -> PID Controller X/1
  PID Controller Y/1 -> Sum8/1
  Sum3/1 -> PID Controller Y/1
  PID Controller X/1 -> Sum7/1
  Sum7/1 -> X'/1
  X/1 -> Sum4/1
  Y/1 -> Sum3/1

== system Quadrotor/Formation Control(PID)/operation ==
  X' : Inport
  Y' : Inport  Port=2
  U1 : Inport  Port=3
  Constant : Constant  Value=m
  Divide : Product  Inputs=*/
  Divide1 : Product  Inputs=*/
  Divide2 : Product  Inputs=*/
  Gain : Gain  Gain=-1
  Product : Product
  Product1 : Product
  Trigonometric Function : Trigonometry  Operator=asin
  Trigonometric Function1 : Trigonometry  Operator=cos
  Trigonometric Function2 : Trigonometry  Operator=asin
  Pitch_d : Outport
  Roll_d : Outport  Port=2
  wires:
  Divide2/1 -> Trigonometric Function2/1
  U1/1 -> Divide1/2, Divide/2
  Divide/1 -> Gain/1
  Trigonometric Function/1 -> Roll_d/1, Trigonometric Function1/1
  Gain/1 -> Trigonometric Function/1
  Trigonometric Function2/1 -> Pitch_d/1
  Trigonometric Function1/1 -> Divide2/2
  Divide1/1 -> Divide2/1
  Product/1 -> Divide1/1
  Product1/1 -> Divide/1
  X'/1 -> Product/1
  Y'/1 -> Product1/2
  Constant/1 -> Product/2, Product1/1

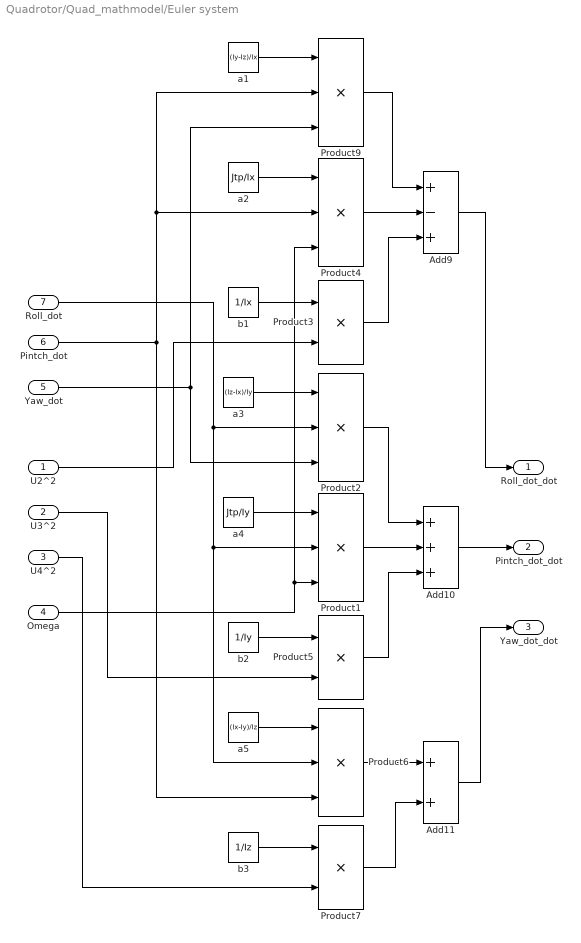
== system Quadrotor/Quad_mathmodel/Euler system ==
  U2^2 : Inport
  U3^2 : Inport  Port=2
  U4^2 : Inport  Port=3
  Omega : Inport  Port=4
  Yaw_dot : Inport  Port=5
  Pintch_dot : Inport  Port=6
  Roll_dot : Inport  Port=7
  Add10 : Sum  Inputs=+++
  Add11 : Sum
  Add9 : Sum  Inputs=+-+
  Product{1..2,4,6,9} (5 alike) : Product  Inputs=3
  Product3 : Product
  Product5 : Product
  Product7 : Product
  a1 : Constant  Value=(Iy-Iz)/Ix
  a2 : Constant  Value=Jtp/Ix
  a3 : Constant  Value=(Iz-Ix)/Iy
  a4 : Constant  Value=Jtp/Iy
  a5 : Constant  Value=(Ix-Iy)/Iz
  b1 : Constant  Value=1/Ix
  b2 : Constant  Value=1/Iy
  b3 : Constant  Value=1/Iz
  Roll_dot_dot : Outport
  Pintch_dot_dot : Outport  Port=2
  Yaw_dot_dot : Outport  Port=3
  wires:
  U2^2/1 -> Product3/2
  Product7/1 -> Add11/2
  Product6/1 -> Add11/1
  Product4/1 -> Add9/2
  Product5/1 -> Add10/3
  a1/1 -> Product9/1
  Add10/1 -> Pintch_dot_dot/1
  a2/1 -> Product4/1
  Pintch_dot/1 -> Product6/3, Product9/2, Product4/2
  Yaw_dot/1 -> Product2/3, Product9/3
  Add11/1 -> Yaw_dot_dot/1
  Product2/1 -> Add10/1
  Omega/1 -> Product4/3, Product1/3
  a5/1 -> Product6/1
  b3/1 -> Product7/1
  a4/1 -> Product1/1
  Roll_dot/1 -> Product2/2, Product1/2, Product6/2
  Product1/1 -> Add10/2
  a3/1 -> Product2/1
  b1/1 -> Product3/1
  Product3/1 -> Add9/3
  b2/1 -> Product5/1
  Product9/1 -> Add9/1
  Add9/1 -> Roll_dot_dot/1
  U3^2/1 -> Product5/2
  U4^2/1 -> Product7/2

== system Quadrotor/Quad_mathmodel/Omega system ==
  U1 : Inport
  U2 : Inport  Port=2
  U3 : Inport  Port=3
  U4 : Inport  Port=4
  Inverse operation : Subsystem
  operation : Subsystem
  U1^2 : Outport
  U2^2 : Outport  Port=2
  U3^2 : Outport  Port=3
  U4^2 : Outport  Port=4
  Omega : Outport  Port=5
  wires:
  Inverse operation/1(U1^2) -> U1^2/1
  Inverse operation/2(U2^2) -> U2^2/1
  Inverse operation/3(U3^2) -> U3^2/1
  Inverse operation/4(U4^2) -> U4^2/1
  Inverse operation/5(Omega) -> Omega/1
  U1/1 -> operation/1(U1)
  U2/1 -> operation/2(U2)
  U3/1 -> operation/3(U3)
  U4/1 -> operation/4(U4)
  operation/1(Omeg1) -> Inverse operation/1(Omeg1)
  operation/2(Omeg2) -> Inverse operation/2(Omeg2)
  operation/3(Omeg3) -> Inverse operation/3(Omeg3)
  operation/4(Omeg4) -> Inverse operation/4(Omeg4)

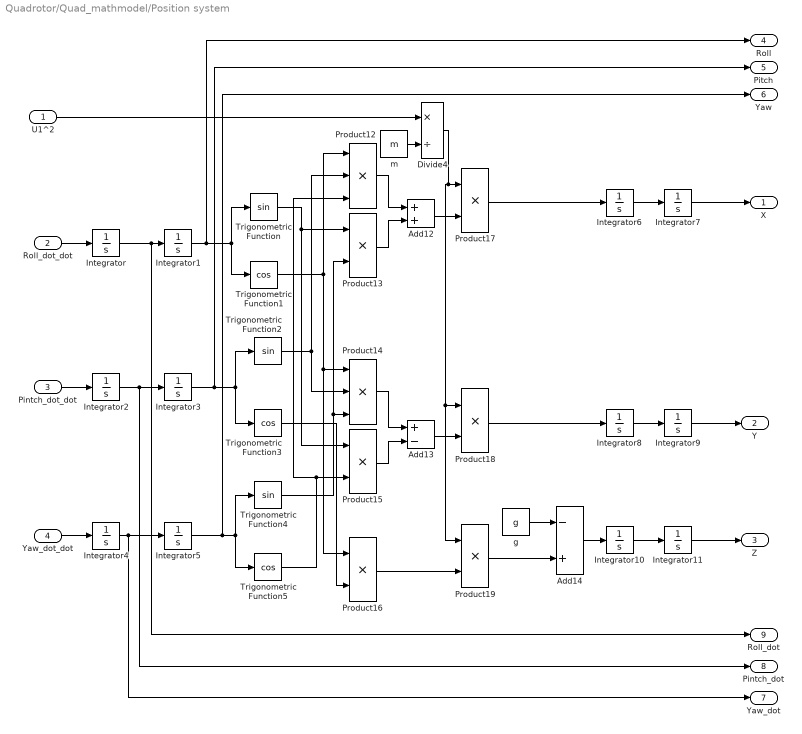
== system Quadrotor/Quad_mathmodel/Position system ==
  U1^2 : Inport
  Roll_dot_dot : Inport  Port=2
  Pintch_dot_dot : Inport  Port=3
  Yaw_dot_dot : Inport  Port=4
  Add12 : Sum
  Add13 : Sum  Inputs=+-
  Add14 : Sum  Inputs=-+
  Divide4 : Product  Inputs=*/
  Integrator{,1..11} (12 alike) : Integrator
  Product12 : Product  Inputs=3
  Product{13,15..19} (6 alike) : Product
  Product14 : Product  Inputs=3
  Trigonometric Function : Trigonometry
  Trigonometric Function1 : Trigonometry  Operator=cos
  Trigonometric Function2 : Trigonometry
  Trigonometric Function3 : Trigonometry  Operator=cos
  Trigonometric Function4 : Trigonometry
  Trigonometric Function5 : Trigonometry  Operator=cos
  g : Constant  Value=g
  m : Constant  Value=m
  X : Outport
  Y : Outport  Port=2
  Z : Outport  Port=3
  Roll : Outport  Port=4
  Pitch : Outport  Port=5
  Yaw : Outport  Port=6
  Yaw_dot : Outport  Port=7
  Pintch_dot : Outport  Port=8
  Roll_dot : Outport  Port=9
  wires:
  Integrator10/1 -> Integrator11/1
  Integrator1/1 -> Roll/1, Trigonometric Function1/1, Trigonometric Function/1
  Trigonometric Function/1 -> Product15/1, Product13/1
  Integrator2/1 -> Pintch_dot/1, Integrator3/1
  Integrator3/1 -> Pitch/1, Trigonometric Function2/1, Trigonometric Function3/1
  Add14/1 -> Integrator10/1
  m/1 -> Divide4/2
  Trigonometric Function1/1 -> Product16/1, Product14/1, Product12/1
  Product19/1 -> Add14/2
  Product15/1 -> Add13/2
  Integrator5/1 -> Yaw/1, Trigonometric Function5/1, Trigonometric Function4/1
  Integrator/1 -> Roll_dot/1, Integrator1/1
  Product16/1 -> Product19/2
  Trigonometric Function2/1 -> Product14/2, Product12/2
  Product14/1 -> Add13/1
  Product13/1 -> Add12/2
  Integrator4/1 -> Yaw_dot/1, Integrator5/1
  Pintch_dot_dot/1 -> Integrator2/1
  Trigonometric Function4/1 -> Product13/2, Product14/3
  g/1 -> Add14/1
  Trigonometric Function5/1 -> Product12/3, Product15/2
  Add12/1 -> Product17/2
  Integrator7/1 -> X/1
  Product12/1 -> Add12/1
  Product18/1 -> Integrator8/1
  Product17/1 -> Integrator6/1
  Add13/1 -> Product18/2
  Roll_dot_dot/1 -> Integrator/1
  Divide4/1 -> Product19/1, Product18/1, Product17/1
  Integrator6/1 -> Integrator7/1
  Integrator8/1 -> Integrator9/1
  Trigonometric Function3/1 -> Product16/2
  Yaw_dot_dot/1 -> Integrator4/1
  U1^2/1 -> Divide4/1
  Integrator9/1 -> Y/1
  Integrator11/1 -> Z/1

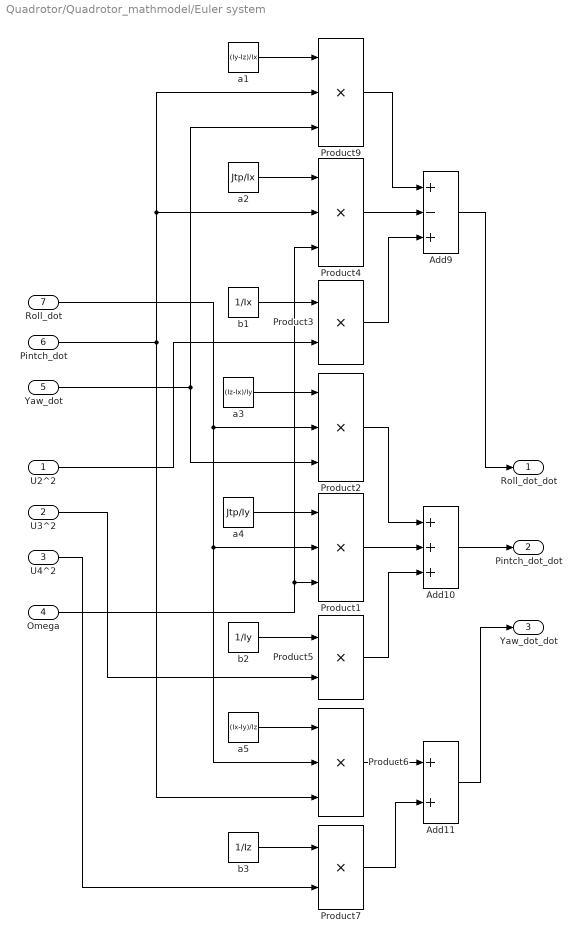
== system Quadrotor/Quadrotor_mathmodel/Euler system ==
  U2^2 : Inport
  U3^2 : Inport  Port=2
  U4^2 : Inport  Port=3
  Omega : Inport  Port=4
  Yaw_dot : Inport  Port=5
  Pintch_dot : Inport  Port=6
  Roll_dot : Inport  Port=7
  Add10 : Sum  Inputs=+++
  Add11 : Sum
  Add9 : Sum  Inputs=+-+
  Product{1..2,4,6,9} (5 alike) : Product  Inputs=3
  Product3 : Product
  Product5 : Product
  Product7 : Product
  a1 : Constant  Value=(Iy-Iz)/Ix
  a2 : Constant  Value=Jtp/Ix
  a3 : Constant  Value=(Iz-Ix)/Iy
  a4 : Constant  Value=Jtp/Iy
  a5 : Constant  Value=(Ix-Iy)/Iz
  b1 : Constant  Value=1/Ix
  b2 : Constant  Value=1/Iy
  b3 : Constant  Value=1/Iz
  Roll_dot_dot : Outport
  Pintch_dot_dot : Outport  Port=2
  Yaw_dot_dot : Outport  Port=3
  wires:
  U2^2/1 -> Product3/2
  Product7/1 -> Add11/2
  Product6/1 -> Add11/1
  Product4/1 -> Add9/2
  Product5/1 -> Add10/3
  a1/1 -> Product9/1
  Add10/1 -> Pintch_dot_dot/1
  a2/1 -> Product4/1
  Pintch_dot/1 -> Product6/3, Product9/2, Product4/2
  Yaw_dot/1 -> Product2/3, Product9/3
  Add11/1 -> Yaw_dot_dot/1
  Product2/1 -> Add10/1
  Omega/1 -> Product4/3, Product1/3
  a5/1 -> Product6/1
  b3/1 -> Product7/1
  a4/1 -> Product1/1
  Roll_dot/1 -> Product2/2, Product1/2, Product6/2
  Product1/1 -> Add10/2
  a3/1 -> Product2/1
  b1/1 -> Product3/1
  Product3/1 -> Add9/3
  b2/1 -> Product5/1
  Product9/1 -> Add9/1
  Add9/1 -> Roll_dot_dot/1
  U3^2/1 -> Product5/2
  U4^2/1 -> Product7/2

== system Quadrotor/Quadrotor_mathmodel/Omega system ==
  U1 : Inport
  U2 : Inport  Port=2
  U3 : Inport  Port=3
  U4 : Inport  Port=4
  Inverse operation : Subsystem
  operation : Subsystem
  U1^2 : Outport
  U2^2 : Outport  Port=2
  U3^2 : Outport  Port=3
  U4^2 : Outport  Port=4
  Omega : Outport  Port=5
  wires:
  Inverse operation/1(U1^2) -> U1^2/1
  Inverse operation/2(U2^2) -> U2^2/1
  Inverse operation/3(U3^2) -> U3^2/1
  Inverse operation/4(U4^2) -> U4^2/1
  Inverse operation/5(Omega) -> Omega/1
  U1/1 -> operation/1(U1)
  U2/1 -> operation/2(U2)
  U3/1 -> operation/3(U3)
  U4/1 -> operation/4(U4)
  operation/1(Omeg1) -> Inverse operation/1(Omeg1)
  operation/2(Omeg2) -> Inverse operation/2(Omeg2)
  operation/3(Omeg3) -> Inverse operation/3(Omeg3)
  operation/4(Omeg4) -> Inverse operation/4(Omeg4)

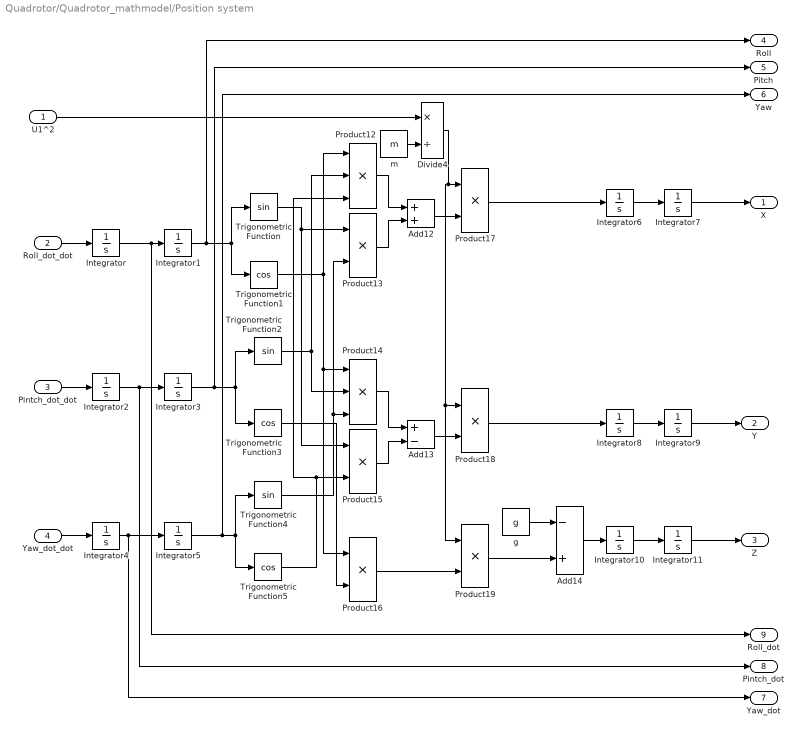
== system Quadrotor/Quadrotor_mathmodel/Position system ==
  U1^2 : Inport
  Roll_dot_dot : Inport  Port=2
  Pintch_dot_dot : Inport  Port=3
  Yaw_dot_dot : Inport  Port=4
  Add12 : Sum
  Add13 : Sum  Inputs=+-
  Add14 : Sum  Inputs=-+
  Divide4 : Product  Inputs=*/
  Integrator{,1..11} (12 alike) : Integrator
  Product12 : Product  Inputs=3
  Product{13,15..19} (6 alike) : Product
  Product14 : Product  Inputs=3
  Trigonometric Function : Trigonometry
  Trigonometric Function1 : Trigonometry  Operator=cos
  Trigonometric Function2 : Trigonometry
  Trigonometric Function3 : Trigonometry  Operator=cos
  Trigonometric Function4 : Trigonometry
  Trigonometric Function5 : Trigonometry  Operator=cos
  g : Constant  Value=g
  m : Constant  Value=m
  X : Outport
  Y : Outport  Port=2
  Z : Outport  Port=3
  Roll : Outport  Port=4
  Pitch : Outport  Port=5
  Yaw : Outport  Port=6
  Yaw_dot : Outport  Port=7
  Pintch_dot : Outport  Port=8
  Roll_dot : Outport  Port=9
  wires:
  Integrator10/1 -> Integrator11/1
  Integrator1/1 -> Roll/1, Trigonometric Function1/1, Trigonometric Function/1
  Trigonometric Function/1 -> Product15/1, Product13/1
  Integrator2/1 -> Pintch_dot/1, Integrator3/1
  Integrator3/1 -> Pitch/1, Trigonometric Function2/1, Trigonometric Function3/1
  Add14/1 -> Integrator10/1
  m/1 -> Divide4/2
  Trigonometric Function1/1 -> Product16/1, Product14/1, Product12/1
  Product19/1 -> Add14/2
  Product15/1 -> Add13/2
  Integrator5/1 -> Yaw/1, Trigonometric Function5/1, Trigonometric Function4/1
  Integrator/1 -> Roll_dot/1, Integrator1/1
  Product16/1 -> Product19/2
  Trigonometric Function2/1 -> Product14/2, Product12/2
  Product14/1 -> Add13/1
  Product13/1 -> Add12/2
  Integrator4/1 -> Yaw_dot/1, Integrator5/1
  Pintch_dot_dot/1 -> Integrator2/1
  Trigonometric Function4/1 -> Product13/2, Product14/3
  g/1 -> Add14/1
  Trigonometric Function5/1 -> Product12/3, Product15/2
  Add12/1 -> Product17/2
  Integrator7/1 -> X/1
  Product12/1 -> Add12/1
  Product18/1 -> Integrator8/1
  Product17/1 -> Integrator6/1
  Add13/1 -> Product18/2
  Roll_dot_dot/1 -> Integrator/1
  Divide4/1 -> Product19/1, Product18/1, Product17/1
  Integrator6/1 -> Integrator7/1
  Integrator8/1 -> Integrator9/1
  Trigonometric Function3/1 -> Product16/2
  Yaw_dot_dot/1 -> Integrator4/1
  U1^2/1 -> Divide4/1
  Integrator9/1 -> Y/1
  Integrator11/1 -> Z/1

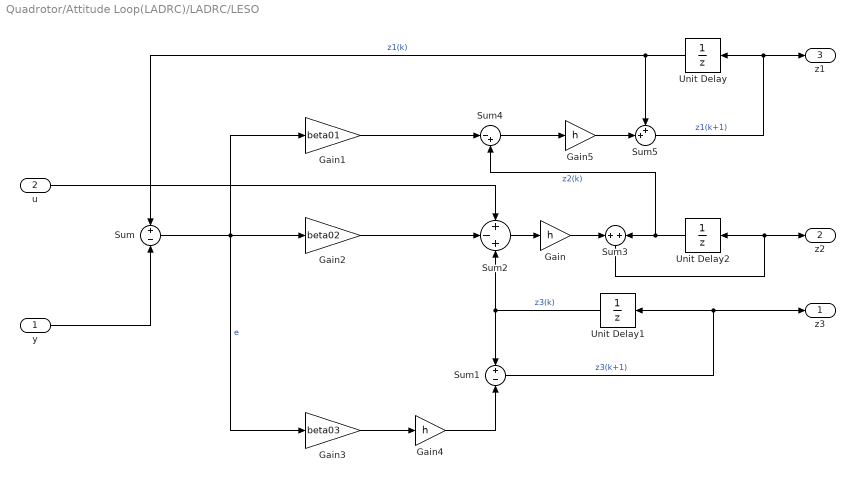
== system Quadrotor/Attitude Loop(LADRC)/LADRC/LESO ==
  y : Inport
  u : Inport  Port=2
  Gain : Gain  Gain=h
  Gain1 : Gain  Gain=beta01
  Gain2 : Gain  Gain=beta02
  Gain3 : Gain  Gain=beta03
  Gain4 : Gain  Gain=h
  Gain5 : Gain  Gain=h
  Sum : Sum  Inputs=+|-
  Sum1 : Sum  Inputs=+-
  Sum2 : Sum  Inputs=+-+
  Sum3 : Sum
  Sum4 : Sum  Inputs=|-+
  Sum5 : Sum  Inputs=++|
  Unit Delay : UnitDelay  SampleTime=-1  HasFrameUpgradeWarning=on
  Unit Delay1 : UnitDelay  SampleTime=-1  HasFrameUpgradeWarning=on
  Unit Delay2 : UnitDelay  SampleTime=-1  HasFrameUpgradeWarning=on
  z3 : Outport
  z2 : Outport  Port=2
  z1 : Outport  Port=3
  wires:
  y/1 -> Sum/2
  Unit Delay/1 -> Sum/1, Sum5/1  "z1(k)"
  Unit Delay1/1 -> Sum2/3, Sum1/1  "z3(k)"
  Sum/1 -> Gain3/1, Gain1/1, Gain2/1  "e"
  Gain3/1 -> Gain4/1
  Gain4/1 -> Sum1/2
  Sum1/1 -> z3/1, Unit Delay1/1  "z3(k+1)"
  Gain2/1 -> Sum2/2
  Sum2/1 -> Gain/1
  Gain/1 -> Sum3/1
  Unit Delay2/1 -> Sum4/2, Sum3/2  "z2(k)"
  Sum3/1 -> Unit Delay2/1, z2/1
  Gain1/1 -> Sum4/1
  Sum4/1 -> Gain5/1
  Gain5/1 -> Sum5/2
  Sum5/1 -> Unit Delay/1, z1/1  "z1(k+1)"
  u/1 -> Sum2/1

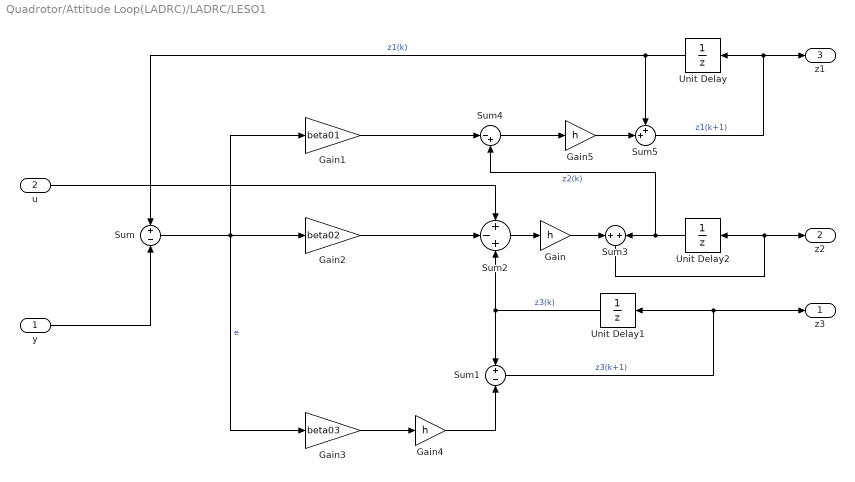
== system Quadrotor/Attitude Loop(LADRC)/LADRC/LESO1 ==
  y : Inport
  u : Inport  Port=2
  Gain : Gain  Gain=h
  Gain1 : Gain  Gain=beta01
  Gain2 : Gain  Gain=beta02
  Gain3 : Gain  Gain=beta03
  Gain4 : Gain  Gain=h
  Gain5 : Gain  Gain=h
  Sum : Sum  Inputs=+|-
  Sum1 : Sum  Inputs=+-
  Sum2 : Sum  Inputs=+-+
  Sum3 : Sum
  Sum4 : Sum  Inputs=|-+
  Sum5 : Sum  Inputs=++|
  Unit Delay : UnitDelay  SampleTime=-1  HasFrameUpgradeWarning=on
  Unit Delay1 : UnitDelay  SampleTime=-1  HasFrameUpgradeWarning=on
  Unit Delay2 : UnitDelay  SampleTime=-1  HasFrameUpgradeWarning=on
  z3 : Outport
  z2 : Outport  Port=2
  z1 : Outport  Port=3
  wires:
  y/1 -> Sum/2
  Unit Delay/1 -> Sum/1, Sum5/1  "z1(k)"
  Unit Delay1/1 -> Sum2/3, Sum1/1  "z3(k)"
  Sum/1 -> Gain3/1, Gain1/1, Gain2/1  "e"
  Gain3/1 -> Gain4/1
  Gain4/1 -> Sum1/2
  Sum1/1 -> z3/1, Unit Delay1/1  "z3(k+1)"
  Gain2/1 -> Sum2/2
  Sum2/1 -> Gain/1
  Gain/1 -> Sum3/1
  Unit Delay2/1 -> Sum4/2, Sum3/2  "z2(k)"
  Sum3/1 -> Unit Delay2/1, z2/1
  Gain1/1 -> Sum4/1
  Sum4/1 -> Gain5/1
  Gain5/1 -> Sum5/2
  Sum5/1 -> Unit Delay/1, z1/1  "z1(k+1)"
  u/1 -> Sum2/1

== system Quadrotor/Attitude Loop(LADRC)/LADRC/LSEF ==
  e1 : Inport
  e2 : Inport  Port=2
  Sum : Sum  Inputs=+-
  kp1 : Gain  Gain=kp1
  kp2 : Gain  Gain=kp2
  u0 : Outport
  wires:
  e1/1 -> kp1/1
  e2/1 -> kp2/1
  kp1/1 -> Sum/1
  kp2/1 -> Sum/2
  Sum/1 -> u0/1

== system Quadrotor/Attitude Loop(LADRC)/LADRC/LSEF1 ==
  e1 : Inport
  e2 : Inport  Port=2
  Sum : Sum
  kp1 : Gain  Gain=kp1
  kp2 : Gain  Gain=kp2
  u0 : Outport
  wires:
  e1/1 -> kp1/1
  e2/1 -> kp2/1
  kp1/1 -> Sum/1
  kp2/1 -> Sum/2
  Sum/1 -> u0/1

== system Quadrotor/Attitude Loop(LADRC)/LADRC/Object ==
  u : Inport
  Integrator : Integrator
  Integrator1 : Integrator  InitialCondition=0.5
  y : Outport
  wires:
  Integrator1/1 -> y/1  "x1"
  Integrator/1 -> Integrator1/1  "x2=dot_x1"
  u/1 -> Integrator/1  "dot_x2"

== system Quadrotor/Attitude Loop(LADRC)/LADRC/Object1 ==
  u : Inport
  Integrator : Integrator
  Integrator1 : Integrator  InitialCondition=0.5
  y : Outport
  wires:
  Integrator1/1 -> y/1  "x1"
  Integrator/1 -> Integrator1/1  "x2=dot_x1"
  u/1 -> Integrator/1  "dot_x2"
